simulink model "Blinking"  (R2016b)
settings: Solver=VariableStepAuto  StartTime=0.0  StopTime=300  RelTol=1e-3
libraries: dspstat3 x1, dspsrcs4 x1
settings Model: Creator=Home  LastModifiedBy=Home

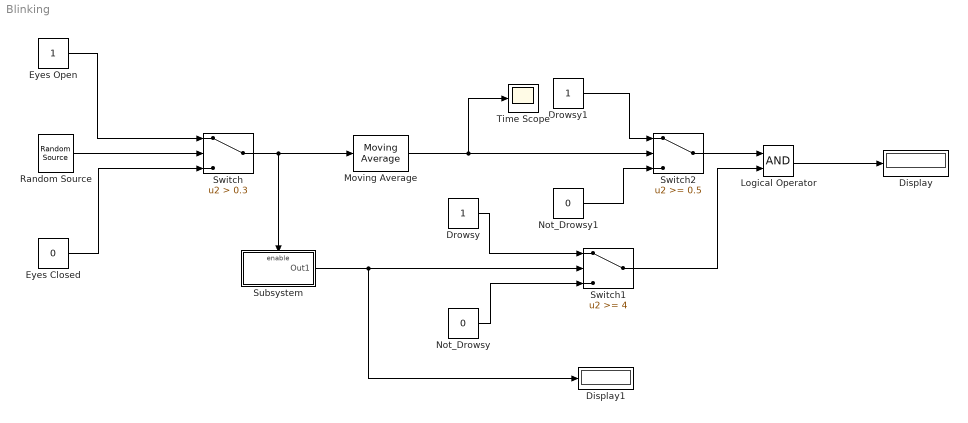
== system Blinking ==
  Display : Display
  Display1 : Display
  Drowsy : Constant
  Drowsy1 : Constant
  Eyes Closed : Constant  Value=0
  Eyes Open : Constant
  Logical Operator : Logic  AllPortsSameDT=off  OutDataTypeStr=boolean
  Moving Average : dspstat3/Moving Average  Method=Sliding window  SpecifyWindowLength=on  WindowLength=30  ForgettingFactor=0.9  SimulateUsing=Code generation
  Not_Drowsy : Constant  Value=0
  Not_Drowsy1 : Constant  Value=0
  Random Source : dspsrcs4/Random Source  SrcType=Uniform  NormMethod=Ziggurat  CltLength=12  MinVal=0  MaxVal=1  MeanVal=0  VarVal=1  RepMode=Repeatable  rawSeed=1  IsInherit=off  SampMode=Discrete  SampTime=0.1  SampFrame=1  DataType=Double  OutComplex=Real  OutputFrames=off
  Subsystem : Subsystem
  Switch : Switch  Criteria=u2 > Threshold  Threshold=0.3
  Switch1 : Switch  Threshold=4
  Switch2 : Switch  Threshold=0.5
  Time Scope : Scope
  wires:
  Random Source/1 -> Switch/2
  Switch/1 -> Moving Average/1, Subsystem/Enable
  Eyes Closed/1 -> Switch/3
  Eyes Open/1 -> Switch/1
  Switch2/1 -> Logical Operator/1
  Logical Operator/1 -> Display/1
  Subsystem/1(Out1) -> Display1/1, Switch1/2
  Not_Drowsy/1 -> Switch1/3
  Drowsy/1 -> Switch1/1
  Switch1/1 -> Logical Operator/2
  Moving Average/1 -> Switch2/2, Time Scope/1
  Not_Drowsy1/1 -> Switch2/3
  Drowsy1/1 -> Switch2/1

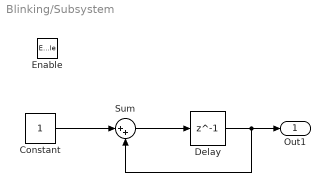
== system Blinking/Subsystem ==
  Enable : EnablePort
  Constant : Constant
  Delay : Delay  DelayLength=1  InitialCondition=0
  Sum : Sum  Inputs=|++
  Out1 : Outport
  wires:
  Delay/1 -> Sum/2, Out1/1
  Sum/1 -> Delay/1
  Constant/1 -> Sum/1
